simulink model "wheelModel"  (R2020b)
settings: Solver=VariableStepAuto  StartTime=0.0  StopTime=4  RelTol=1e-3
settings Model: Creator=lemck  LastModifiedBy=lemck

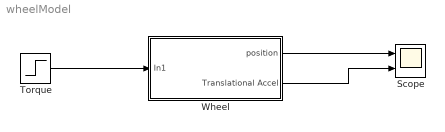
== system wheelModel ==
  Scope : Scope  NumInputPorts=2
  Torque : Step  After=0.05  SampleTime=0
  Wheel : Subsystem
  wires:
  Torque/1 -> Wheel/1(In1)
  Wheel/1(position) -> Scope/1
  Wheel/2(Translational Accel) -> Scope/2

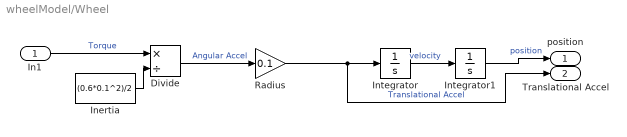
== system wheelModel/Wheel ==
  In1 : Inport
  Divide : Product  Inputs=*/
  Inertia : Constant  Value=(0.6*0.1^2)/2
  Integrator : Integrator
  Integrator1 : Integrator
  Radius : Gain  Gain=0.1
  position : Outport
  Translational Accel : Outport  Port=2
  wires:
  Divide/1 -> Radius/1  "Angular Accel"
  Inertia/1 -> Divide/2
  Integrator/1 -> Integrator1/1  "velocity"
  Radius/1 -> Translational Accel/1, Integrator/1  "Translational Accel"
  In1/1 -> Divide/1  "Torque"
  Integrator1/1 -> position/1  "position"
